simulink model "link_type"  (R2014a)
settings: Solver=ode45  StartTime=0.0  StopTime=10.0  RelTol=1e-3
settings Model: Creator=ehb9kor  LastModifiedBy=ladmin
settings DebuggingCC: UnderspecifiedInitializationDetection=Classic  FcnCallInpInsideContextMsg=EnableAllAsWarning
settings GRTTargetCC: CombineOutputUpdateFcns=off  GRTInterface=on

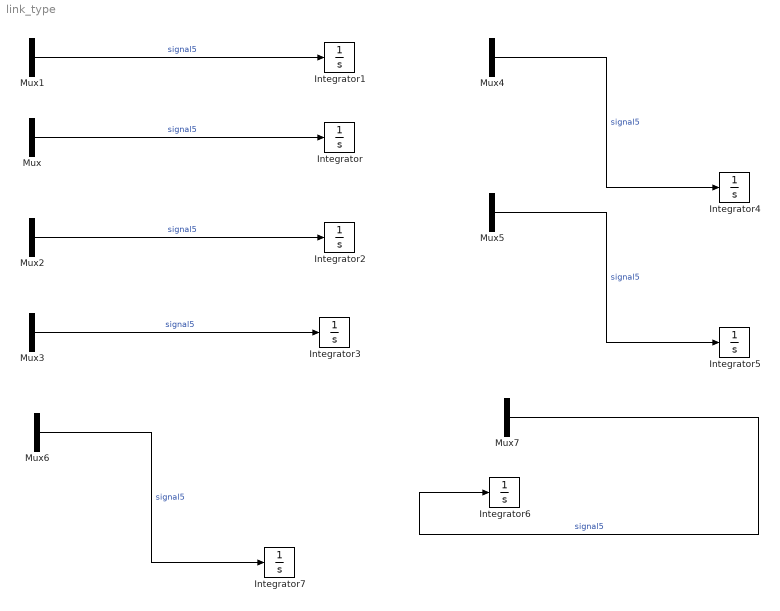
== system link_type ==
  Integrator{,1..7} (8 alike) : Integrator
  Mux{,1..7} (8 alike) : Mux  Inputs=2
  wires:
  Mux/1 -> Integrator/1  "signal5"
  Mux1/1 -> Integrator1/1  "signal5"
  Mux3/1 -> Integrator3/1  "signal5"
  Mux4/1 -> Integrator4/1  "signal5"
  Mux5/1 -> Integrator5/1  "signal5"
  Mux6/1 -> Integrator7/1  "signal5"
  Mux7/1 -> Integrator6/1  "signal5"
  Mux2/1 -> Integrator2/1  "signal5"
